simulink model "PV_MEV"  (R2025a)
settings: Solver=VariableStepAuto  StartTime=0.0  StopTime=10.0  RelTol=1e-3
InitFcn:
  | init_paras
values from neighbouring files (symbols this model uses):
  C_PFC = 2600e-6    (= 0.0026)    [init_paras.m]
  chg_ctrl_par = [Icc Vcv V_hys T_hys Kp_v_chg Ki_v_chg Kp_i_chg Ki_i_chg Ts_chg D_max_chg t_chg_on k_chg]    [init_paras.m]
  chg_ev = [0 Icc]    [init_paras.m]
  chg_par = [L_chg Voc Rint Ts_chg I_SIGN t_chg_on]    [init_paras.m]
  D = struct('X', {}, 'ti', {}, 'ia', {}, 'tc', {}, 'irms', {}, 'thd', {}, 'trip', {}, 'ttrip', {})    [make_waveform_figs.m]    (also in run_benchmark.m = get_sig('D'))
  det_ema_alpha = 0.1    [init_paras.m]
  det_force = 0    [init_paras.m]
  det_hyst = 0.6    [init_paras.m]
  det_persist = 2    [init_paras.m]
  det_src = 0    [init_paras.m]
  det_t_arm = 0.58    [init_paras.m]
  det_thr = [0.5 0.5 0.5 0.5 0.5]    [init_paras.m]
  det_variant_onehot = double(det_vlist == VARIANT_NAME)    [init_paras.m]
  ENABLE_HIL = 0    [init_paras.m]
  ENABLE_HIL_DET = 0    [init_paras.m]
  ENABLE_HIL_EST = 0    [init_paras.m]
  estimation_src = cfg_row.estimation_src    [init_paras.m]
  Fnom = 50    [init_paras.m]
  Fr_I = Fnom*2    (= 100)    [init_paras.m]
  grid_df = 0    [init_paras.m]
  grid_h5 = 0    [init_paras.m]
  grid_h7 = 0    [init_paras.m]
  grid_var_t0 = 0.7    [init_paras.m]
  hgq_fusion_alpha = [0.6704476522845647 0.7221651725151749 0.6446423751787858 0.41926421682656173]    [init_paras.m]
  hgq_min_ratio = single(0)    [init_paras.m]
  inj_channel = INJ.channel    [init_paras.m]
  inj_dwell = INJ.dwell    [init_paras.m]
  inj_shape = INJ.shape    [init_paras.m]
  inj_t_on = INJ.t_on    [init_paras.m]
  Ki_V = 80    [init_paras.m]
  Kp_I = 0.06    [init_paras.m]
  Kp_V = 0.25    [init_paras.m]
  Kr_I = 2.5    [init_paras.m]
  L_PFC = 600e-6    (= 0.0006)    [init_paras.m]
  Limit_V = 100    [init_paras.m]
  mit_t_ramp = 0.06    [init_paras.m]
  mitigation_mask = 0    [init_paras.m]
  mm_10cycle_points = mm_points_per_cycle * 10    (= 800)    [init_paras.m]
  mm_fund_freq = 50    [init_paras.m]
  mm_points_per_cycle = 80    [init_paras.m]
  R_bleed = 100e3    (= 100000)    [init_paras.m]
  R_pre = Ro*2    (= 44.44)    [init_paras.m]
  res_par = double(RES.par(:)'); end    [init_paras.m]
  RL_PFC = 20e-3    (= 0.02)    [init_paras.m]
  Ro = 22.22    [init_paras.m]
  t_pre_off = 0.30    (= 0.3)    [init_paras.m]
  Ts_chg = 10e-6    (= 1e-05)    [init_paras.m]
  Ts_Control = 1/Fc    [init_paras.m]
  Ts_Power = 50e-9    (= 5e-08)    [init_paras.m]    (also in run_benchmark.m = evalin('base','Ts_Power'))
  use_d_predict = cfg_row.use_d_predict    [init_paras.m]
  use_detector = 0    [init_paras.m]
  use_harmonic = cfg_row.use_harmonic    [init_paras.m]
  use_p_predict = cfg_row.use_p_predict    [init_paras.m]
  Vnom_ac = 240    [init_paras.m]
  vref_ev = [0 0]    [init_paras.m]
undefined symbols (not defined in the file or in its folder): D1, Delta, DiscIntNeverNeededParam
libraries: spsSeriesRLCBranchLib x17, spsMeanLib x16, MyLibrary x12, spsCurrentMeasurementLib x9, spsFourierLib x8, spsTHDLib x8, spsVoltageMeasurementLib x8, spsDiodeLib x7, simulink x7, pycoexlib x5, instrumentlib x4, spsPWMGeneratorDCDCLib x4
(part 3 of 7)

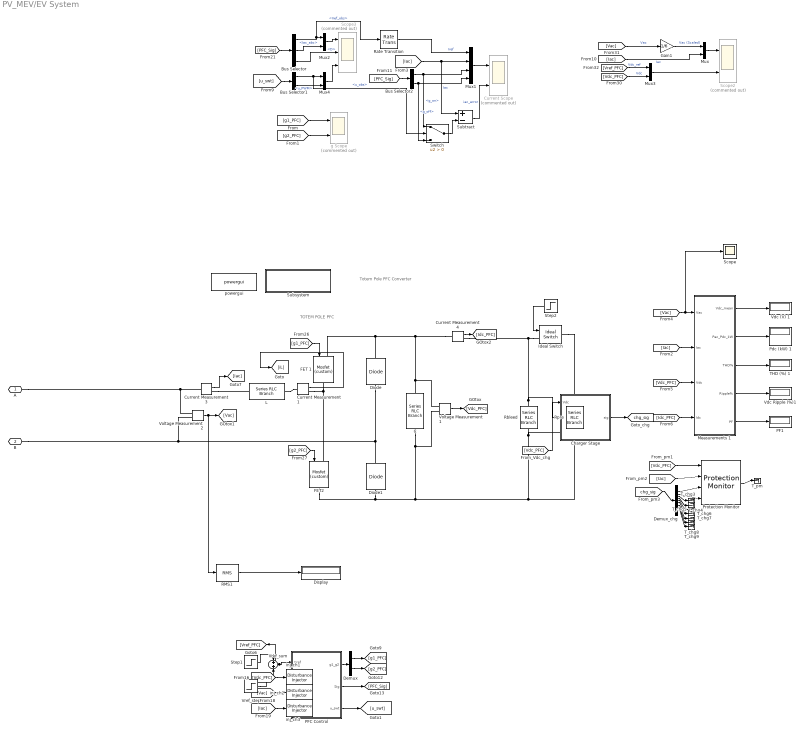
== system PV_MEV/EV System ==
  note: TOTEM POLE PFC
  note: Totem Pole PFC Converter
  Bus Selector : BusSelector  OutputSignals=Iref_obs,Iac_abc,D
  Bus Selector1 : BusSelector  OutputSignals=u_obs,u_PWM
  Bus Selector2 : BusSelector  OutputSignals=g_on,g_off
  C : spsSeriesRLCBranchLib/Series RLC Branch  LConnTagsString=__new0  RConnTagsString=__new0  BranchType=C  Resistance=1  Inductance=1e-3  SetiL0=off  InitialCurrent=0  Capacitance=C_PFC  Setx0=on  InitialVoltage=375  Measurements=None
  Charger Stage : Subsystem  mask(Charger Stage){}
      mask Display: disp('charger\\nbuck + battery\\nCC/CV')
  Current Measurement1 : spsCurrentMeasurementLib/Current Measurement  PhasorSimulation=off  OutputType=Complex  PSBequivalent=0
  Current Measurement3 : spsCurrentMeasurementLib/Current Measurement  PhasorSimulation=off  OutputType=Complex  PSBequivalent=0
  Current Measurement4 : spsCurrentMeasurementLib/Current Measurement  PhasorSimulation=off  OutputType=Complex  PSBequivalent=0
  Current Scope : Scope  Commented=on  NumInputPorts=2
      settings: ActiveDisplayYMinimum=-76.3871  ActiveDisplayYMaximum=79.5142  DataLoggingSaveFormat=Array
  Demux : Demux  Outputs=2
  Demux_chg : Demux  Outputs=9
  Diode : spsDiodeLib/Diode  Ron=Ron_Diode  Lon=0  Vf=Vf  IC=0  UseSnubber=0  Rs=1e6  Cs=inf  Measurements=off
  Diode1 : spsDiodeLib/Diode  Ron=Ron_Diode  Lon=0  Vf=Vf  IC=0  UseSnubber=0  Rs=1e6  Cs=inf  Measurements=off
  Display : Display
  FET 1 : MyLibrary/Mosfet (custom)  Ron=Ron_FET  Lon=0  Rd=Ron_Diode  Vfd=Vf  IC=0  Rs=1e6  Cs=inf  Measurements=off
  FET2 : MyLibrary/Mosfet (custom)  Ron=Ron_FET  Lon=0  Rd=Ron_Diode  Vfd=Vf  IC=0  Rs=1e6  Cs=inf  Measurements=off
  Gain1 : Gain  Gain=1/6
  Ideal Switch : spsIdealSwitchLib/Ideal Switch  Ron=0.001  Lon=0  IC=0  Rs=1e5  Cs=inf  Measurements=off
  L : spsSeriesRLCBranchLib/Series RLC Branch  LConnTagsString=__new0  RConnTagsString=__new0  BranchType=RL  Resistance=RL_PFC  Inductance=L_PFC  SetiL0=off  InitialCurrent=0  Capacitance=1e-6  Setx0=off  InitialVoltage=0  Measurements=None
  Measurements 1 : Subsystem
  Mux{,2..4} (4 alike) : Mux  Inputs=2
  Mux1 : Mux
  PF1 : Display
      settings: Format=bank  Decimation=100
  PFC Control : Subsystem
  Pdc (kW) 1 : Display
      settings: Format=bank  Decimation=100
  Protection Monitor : MyLibrary/Protection Monitor  SystemSampleTime=-1  VariantActivationTime=update diagram  EmptyChoice=off  PassThrough=off  PassThroughVariantControl=(default)  EmptyChoiceVariantControl=(default)  AllowFlexibleInterface=on  Latency=0  AutoFrameSizeCalculation=off
  RMS1 : spsRMSLib/RMS  TrueRMS=on  Freq=60  RMSInit=0  Ts=5E-08
  Rate Transition : RateTransition
  Rbleed : spsSeriesRLCBranchLib/Series RLC Branch  LConnTagsString=__new0  RConnTagsString=__new0  BranchType=R  Resistance=R_bleed  Inductance=200e-6  SetiL0=off  InitialCurrent=0  Capacitance=400e-6  Setx0=off  InitialVoltage=0  Measurements=None
  Rpre : spsSeriesRLCBranchLib/Series RLC Branch  LConnTagsString=__new0  RConnTagsString=__new0  BranchType=R  Resistance=R_pre  Inductance=200e-6  SetiL0=off  InitialCurrent=0  Capacitance=400e-6  Setx0=off  InitialVoltage=0  Measurements=None
  Scope : Scope
      settings: ActiveDisplayYMaximum=209.9376  DataLoggingVariableName=ScopeData2  DataLoggingSaveFormat=Array
  Scope2 : Scope  Commented=on  NumInputPorts=2
      settings: ActiveDisplayYMinimum=-127.2219  ActiveDisplayYMaximum=127.2109  DataLoggingVariableName=ScopeData3  DataLoggingSaveFormat=Array
  Scope3 : Scope  Commented=on  NumInputPorts=3
      settings: ActiveDisplayYMinimum=-13.4274  ActiveDisplayYMaximum=110.8467  DataLoggingVariableName=ScopeData4  DataLoggingSaveFormat=Array
  Step1 : Step  Time=0.2  Before=350  After=400  SampleTime=Ts_Power
  Step2 : Step  Time=t_pre_off  Before=1  After=0  SampleTime=Ts_Power
  Subsystem : Subsystem
      settings: OpenFcn=edit('Totem_Pole_PFC_v1_data');
      mask Display: disp('Double-click to open\n parameters file');
  Subtract : Sum  Inputs=+-
  Switch : Switch  Criteria=u2 > Threshold  SaturateOnIntegerOverflow=off  InputSameDT=off
  THD (%) 1 : Display
      settings: Format=bank  Decimation=100
  T_chg{3..9} (7 alike) : Terminator
  T_pm : Terminator
  Vdc (V) 1 : Display
      settings: Format=bank  Decimation=100
  Vdc Ripple (%)1 : Display
      settings: Format=bank  Decimation=100
  Voltage Measurement1 : spsVoltageMeasurementLib/Voltage Measurement  PhasorSimulation=off  OutputType=Complex  PSBequivalent=0
  Voltage Measurement2 : spsVoltageMeasurementLib/Voltage Measurement  PhasorSimulation=off  OutputType=Complex  PSBequivalent=0
  Vref_step : Step  Time=vref_ev(1)  After=vref_ev(2)  SampleTime=0
  Vref_sum : Sum
  g Scope : Scope  Commented=on  NumInputPorts=2
      settings: ActiveDisplayYMinimum=-0.125  ActiveDisplayYMaximum=1.125  DataLoggingVariableName=ScopeData5  DataLoggingSaveFormat=Array
  inj_ch1 : MyLibrary/Disturbance Injector  ch_id=1  Ts_inj=Ts_Control  Ts_out=Ts_Power
  inj_ch2 : MyLibrary/Disturbance Injector  ch_id=2  Ts_inj=Ts_Control  Ts_out=Ts_Power
  inj_ch3 : MyLibrary/Disturbance Injector  ch_id=3  Ts_inj=Ts_Control  Ts_out=Ts_Power
  powergui : spspowerguiLib/powergui  Priority=1  SimulationMode=Discrete  SampleTime=Ts_Power  frequency=60  Iterations=50  frequencyindice=0  Pbase=100e6  ErrMax=1e-4  UnitsV=kV  UnitsW=MW  buscounter=0  FunctionMessages=off  echomessages=off  EnableUseOfTLC=off  CurrentSourceSwitches=off  DisableSnubberDevices=off  DisableRonSwitches=off  DisableVfSwitches=off  DisplayEquations=off  AutomaticDiscreteSolvers=off  SolverType=Tustin/Backward Euler (TBE)  Interpol=off  ExternalGateDelay=off  methode=off  Ts=100  x0status=blocks  SPID=on  SwTol=0  HookPort=off  NonlinearTolerance=1e-4  nMaxIteration=100  ContinueOnMaxIteration=off  RestoreLinks=warning  ResistiveCurrentMeasurement=off  Frange=[0:2:500]  Ylog=off  Xlog=on  ShowGrid=off  save=off  variable=ZData  structure=0  ZoomFFT=off  StartTime=0.0  cycles=1  DisplayStyle=1  fundamental=60  FreqAxis=off  MaxFrequency=1000  frequencyindicesteady=1  RmsSteady=1  display=off
  A : PMIOPort  Side=Left
  B : PMIOPort  Port=2  Side=Left
  tag scope: chg_sig=global
  wires:
  Bus Selector1/1 -> Mux4/1, Switch/2  "<u_obs>"
  Bus Selector/2 -> Mux2/2  "<Iac_abc>"
  [g2_PFC] -> FET2/1
  [Iac] -> Measurements 1/2(Iac)
  Bus Selector/3 -> Scope3/2  "<D>"
  [g1_PFC] -> g Scope/1
  Measurements 1/3(THD%) -> THD (%) 1/1
  Voltage Measurement2/1 -> RMS1/1, [Vac]
  Mux3/1 -> Scope2/2
  Measurements 1/4(Ripple%) -> Vdc Ripple (%)1/1
  PFC Control/1(g1_g2) -> Demux/1
  PFC Control/3(u_swt) -> [u_swt]
  Bus Selector2/2 -> Mux1/4, Switch/3  "<g_off>"
  Mux2/1 -> Scope3/1
  Measurements 1/2(Pac_Pdc_kW) -> Pdc (kW) 1/1
  Step2/1 -> Ideal Switch/1
  [Idc_PFC] -> Measurements 1/4(Idc)
  [Iac] -> Subtract/1, Mux1/2  "Iac"
  Gain1/1 -> Mux/1  "Vac (Scaled)"
  [u_swt] -> Bus Selector1/1
  Bus Selector/1 -> Rate Transition/1, Mux2/1  "<Iref_obs>"
  Measurements 1/1(Vdc_mean) -> Vdc (V) 1/1
  [g2_PFC] -> g Scope/2
  [PFC_Sig] -> Bus Selector2/1
  [Vac] -> Scope/1, Measurements 1/1(Vac)
  [Vac] -> Gain1/1  "Vac"
  PFC Control/2(Sig) -> [PFC_Sig]
  [PFC_Sig] -> Bus Selector/1
  Voltage Measurement1/1 -> [Vdc_PFC]
  [g1_PFC] -> FET 1/1
  [Vdc_PFC] -> Measurements 1/3(Vdc)
  Mux/1 -> Scope2/1
  Bus Selector1/2 -> Mux4/2  "<u_PWM>"
  RMS1/1 -> Display/1
  Current Measurement3/1 -> [Iac]
  [Iac] -> Mux/2  "Iac"
  Bus Selector2/1 -> Switch/1, Mux1/3  "<g_on>"
  Switch/1 -> Subtract/2
  Current Measurement1/1 -> [iL]
  Mux4/1 -> Scope3/3
  [Vdc_PFC] -> Mux3/2  "Vdc"
  Demux/1 -> [g1_PFC]
  Demux/2 -> [g2_PFC]
  Rate Transition/1 -> Mux1/1  "Iref"
  Measurements 1/5(PF) -> PF1/1
  Mux1/1 -> Current Scope/1
  [Vref_PFC] -> Mux3/1  "Vdc_ref"
  Subtract/1 -> Current Scope/2  "iac_error"
  Current Measurement4/1 -> [Idc_PFC]
  [Vdc_PFC] -> Charger Stage/1(Vdc)
  Charger Stage/1(sig) -> [chg_sig]
  [Vdc_PFC] -> inj_ch1/1
  inj_ch1/1 -> PFC Control/2(Vdc)
  [Vac] -> inj_ch2/1
  inj_ch2/1 -> PFC Control/3(Vac)
  [Iac] -> inj_ch3/1
  inj_ch3/1 -> PFC Control/4(Iac)
  [Vdc_PFC] -> Protection Monitor/1
  [Iac] -> Protection Monitor/2
  [chg_sig] -> Demux_chg/1
  Demux_chg/1 -> Protection Monitor/3
  Demux_chg/2 -> Protection Monitor/4
  Demux_chg/3 -> T_chg3/1
  Demux_chg/4 -> T_chg4/1
  Demux_chg/5 -> T_chg5/1
  Demux_chg/6 -> T_chg6/1
  Demux_chg/7 -> T_chg7/1
  Demux_chg/8 -> T_chg8/1
  Demux_chg/9 -> T_chg9/1
  Protection Monitor/1 -> T_pm/1
  Step1/1 -> Vref_sum/1
  Vref_step/1 -> Vref_sum/2
  Vref_sum/1 -> PFC Control/1(Vref), [Vref_PFC]
  connections:
  Ideal Switch/LConn1 -- Current Measurement4/RConn1 -- Rbleed/LConn1 -- Charger Stage/LConn1
  Current Measurement1/RConn1 -- FET2/LConn1 -- FET 1/RConn1
  Rpre/RConn1 -- Rbleed/RConn1 -- Charger Stage/LConn2 -- C/RConn1 -- Voltage Measurement1/LConn2 -- FET2/RConn1 -- Diode1/LConn1
  Voltage Measurement2/LConn2 -- B/RConn1 -- Diode/LConn1 -- Diode1/RConn1
  Current Measurement4/LConn1 -- Voltage Measurement1/LConn1 -- C/LConn1 -- Diode/RConn1 -- FET 1/LConn1
  Voltage Measurement2/LConn1 -- A/RConn1 -- Current Measurement3/LConn1
  Current Measurement3/RConn1 -- L/LConn1
  L/RConn1 -- Current Measurement1/LConn1
  Ideal Switch/RConn1 -- Rpre/LConn1

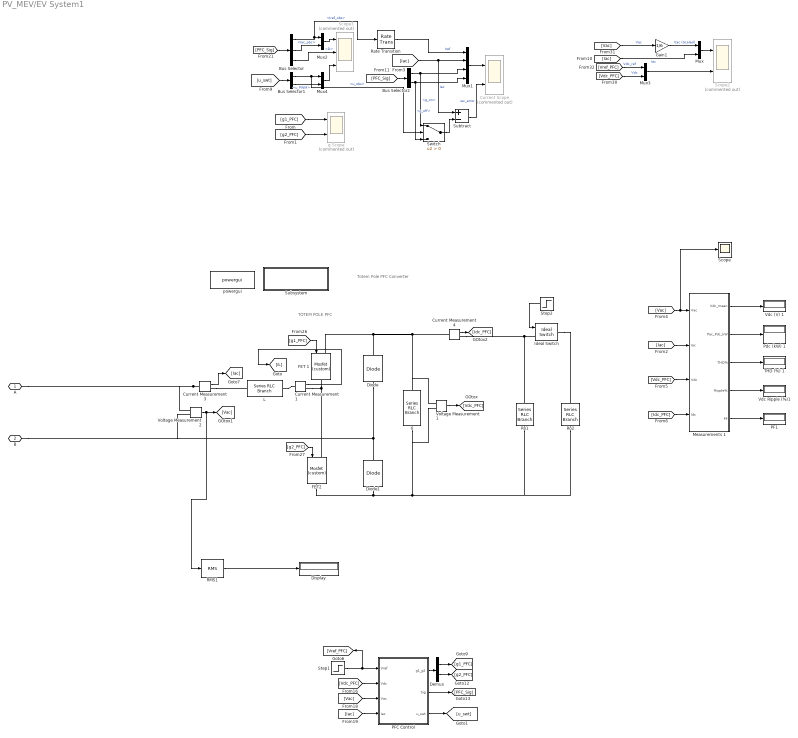
== system PV_MEV/EV System1 ==
  note: Totem Pole PFC Converter
  note: TOTEM POLE PFC
  Bus Selector : BusSelector  OutputSignals=Iref_obs,Iac_abc,D
  Bus Selector1 : BusSelector  OutputSignals=u_obs,u_PWM
  Bus Selector2 : BusSelector  OutputSignals=g_on,g_off
  C : spsSeriesRLCBranchLib/Series RLC Branch  LConnTagsString=__new0  RConnTagsString=__new0  BranchType=C  Resistance=1  Inductance=1e-3  SetiL0=off  InitialCurrent=0  Capacitance=C_PFC  Setx0=on  InitialVoltage=375  Measurements=None
  Current Measurement1 : spsCurrentMeasurementLib/Current Measurement  PhasorSimulation=off  OutputType=Complex  PSBequivalent=0
  Current Measurement3 : spsCurrentMeasurementLib/Current Measurement  PhasorSimulation=off  OutputType=Complex  PSBequivalent=0
  Current Measurement4 : spsCurrentMeasurementLib/Current Measurement  PhasorSimulation=off  OutputType=Complex  PSBequivalent=0
  Current Scope : Scope  Commented=on  NumInputPorts=2
      settings: ActiveDisplayYMinimum=-76.3871  ActiveDisplayYMaximum=79.5142  DataLoggingSaveFormat=Array
  Demux : Demux  Outputs=2
  Diode : spsDiodeLib/Diode  Ron=Ron_Diode  Lon=0  Vf=Vf  IC=0  UseSnubber=0  Rs=1e6  Cs=inf  Measurements=off
  Diode1 : spsDiodeLib/Diode  Ron=Ron_Diode  Lon=0  Vf=Vf  IC=0  UseSnubber=0  Rs=1e6  Cs=inf  Measurements=off
  Display : Display
  FET 1 : MyLibrary/Mosfet (custom)  Ron=Ron_FET  Lon=0  Rd=Ron_Diode  Vfd=Vf  IC=0  Rs=1e6  Cs=inf  Measurements=off
  FET2 : MyLibrary/Mosfet (custom)  Ron=Ron_FET  Lon=0  Rd=Ron_Diode  Vfd=Vf  IC=0  Rs=1e6  Cs=inf  Measurements=off
  Gain1 : Gain  Gain=1/6
  Ideal Switch : spsIdealSwitchLib/Ideal Switch  Ron=0.001  Lon=0  IC=0  Rs=1e5  Cs=inf  Measurements=off
  L : spsSeriesRLCBranchLib/Series RLC Branch  LConnTagsString=__new0  RConnTagsString=__new0  BranchType=RL  Resistance=RL_PFC  Inductance=L_PFC  SetiL0=off  InitialCurrent=0  Capacitance=1e-6  Setx0=off  InitialVoltage=0  Measurements=None
  Measurements 1 : Subsystem
  Mux{,2..4} (4 alike) : Mux  Inputs=2
  Mux1 : Mux
  PF1 : Display
      settings: Format=bank  Decimation=100
  PFC Control : Subsystem
  Pdc (kW) 1 : Display
      settings: Format=bank  Decimation=100
  RMS1 : spsRMSLib/RMS  TrueRMS=on  Freq=60  RMSInit=0  Ts=5E-08
  Rate Transition : RateTransition
  Ro1 : spsSeriesRLCBranchLib/Series RLC Branch  LConnTagsString=__new0  RConnTagsString=__new0  BranchType=R  Resistance=Ro*2  Inductance=200e-6  SetiL0=off  InitialCurrent=0  Capacitance=400e-6  Setx0=off  InitialVoltage=0  Measurements=None
  Ro2 : spsSeriesRLCBranchLib/Series RLC Branch  LConnTagsString=__new0  RConnTagsString=__new0  BranchType=R  Resistance=Ro*2  Inductance=200e-6  SetiL0=off  InitialCurrent=0  Capacitance=400e-6  Setx0=off  InitialVoltage=0  Measurements=None
  Scope : Scope
      settings: DataLoggingVariableName=ScopeData2  DataLoggingSaveFormat=Array
  Scope2 : Scope  Commented=on  NumInputPorts=2
      settings: ActiveDisplayYMinimum=-127.2219  ActiveDisplayYMaximum=127.2109  DataLoggingVariableName=ScopeData3  DataLoggingSaveFormat=Array
  Scope3 : Scope  Commented=on  NumInputPorts=3
      settings: ActiveDisplayYMinimum=-13.4274  ActiveDisplayYMaximum=110.8467  DataLoggingVariableName=ScopeData4  DataLoggingSaveFormat=Array
  Step1 : Step  Time=0.2  Before=350  After=400  SampleTime=Ts_Power
  Step2 : Step  Time=0.4  SampleTime=Ts_Power
  Subsystem : Subsystem
      settings: OpenFcn=edit('Totem_Pole_PFC_v1_data');
      mask Display: disp('Double-click to open\n parameters file');
  Subtract : Sum  Inputs=+-
  Switch : Switch  Criteria=u2 > Threshold  SaturateOnIntegerOverflow=off  InputSameDT=off
  THD (%) 1 : Display
      settings: Format=bank  Decimation=100
  Vdc (V) 1 : Display
      settings: Format=bank  Decimation=100
  Vdc Ripple (%)1 : Display
      settings: Format=bank  Decimation=100
  Voltage Measurement1 : spsVoltageMeasurementLib/Voltage Measurement  PhasorSimulation=off  OutputType=Complex  PSBequivalent=0
  Voltage Measurement2 : spsVoltageMeasurementLib/Voltage Measurement  PhasorSimulation=off  OutputType=Complex  PSBequivalent=0
  g Scope : Scope  Commented=on  NumInputPorts=2
      settings: ActiveDisplayYMinimum=-0.125  ActiveDisplayYMaximum=1.125  DataLoggingVariableName=ScopeData5  DataLoggingSaveFormat=Array
  powergui : spspowerguiLib/powergui  Priority=1  SimulationMode=Discrete  SampleTime=Ts_Power  frequency=60  Iterations=50  frequencyindice=0  Pbase=100e6  ErrMax=1e-4  UnitsV=kV  UnitsW=MW  buscounter=0  FunctionMessages=off  echomessages=off  EnableUseOfTLC=off  CurrentSourceSwitches=off  DisableSnubberDevices=off  DisableRonSwitches=off  DisableVfSwitches=off  DisplayEquations=off  AutomaticDiscreteSolvers=off  SolverType=Tustin/Backward Euler (TBE)  Interpol=off  ExternalGateDelay=off  methode=off  Ts=100  x0status=blocks  SPID=on  SwTol=0  HookPort=off  NonlinearTolerance=1e-4  nMaxIteration=100  ContinueOnMaxIteration=off  RestoreLinks=warning  ResistiveCurrentMeasurement=off  Frange=[0:2:500]  Ylog=off  Xlog=on  ShowGrid=off  save=off  variable=ZData  structure=0  ZoomFFT=off  StartTime=0.0  cycles=1  DisplayStyle=1  fundamental=60  FreqAxis=off  MaxFrequency=1000  frequencyindicesteady=1  RmsSteady=1  display=off
  A : PMIOPort  Side=Left
  B : PMIOPort  Port=2  Side=Left
  wires:
  Current Measurement4/1 -> [Idc_PFC]
  Subtract/1 -> Current Scope/2  "iac_error"
  [Vref_PFC] -> Mux3/1  "Vdc_ref"
  Mux1/1 -> Current Scope/1
  Measurements 1/5(PF) -> PF1/1
  Rate Transition/1 -> Mux1/1  "Iref"
  Demux/2 -> [g2_PFC]
  Demux/1 -> [g1_PFC]
  [Vdc_PFC] -> Mux3/2  "Vdc"
  Mux4/1 -> Scope3/3
  [Iac] -> PFC Control/4(Iac)
  Current Measurement1/1 -> [iL]
  Switch/1 -> Subtract/2
  Bus Selector2/1 -> Mux1/3, Switch/1  "<g_on>"
  [Iac] -> Mux/2  "Iac"
  Current Measurement3/1 -> [Iac]
  RMS1/1 -> Display/1
  Bus Selector1/2 -> Mux4/2  "<u_PWM>"
  Mux/1 -> Scope2/1
  [Vdc_PFC] -> Measurements 1/3(Vdc)
  [Vac] -> PFC Control/3(Vac)
  [g1_PFC] -> FET 1/1
  Voltage Measurement1/1 -> [Vdc_PFC]
  [Vdc_PFC] -> PFC Control/2(Vdc)
  [PFC_Sig] -> Bus Selector/1
  PFC Control/2(Sig) -> [PFC_Sig]
  [Vac] -> Gain1/1  "Vac"
  [Vac] -> Measurements 1/1(Vac), Scope/1
  [PFC_Sig] -> Bus Selector2/1
  [g2_PFC] -> g Scope/2
  Measurements 1/1(Vdc_mean) -> Vdc (V) 1/1
  Bus Selector/1 -> Mux2/1, Rate Transition/1  "<Iref_obs>"
  [u_swt] -> Bus Selector1/1
  Gain1/1 -> Mux/1  "Vac (Scaled)"
  [Iac] -> Mux1/2, Subtract/1  "Iac"
  [Idc_PFC] -> Measurements 1/4(Idc)
  Step2/1 -> Ideal Switch/1
  Measurements 1/2(Pac_Pdc_kW) -> Pdc (kW) 1/1
  Mux2/1 -> Scope3/1
  Bus Selector2/2 -> Switch/3, Mux1/4  "<g_off>"
  PFC Control/3(u_swt) -> [u_swt]
  PFC Control/1(g1_g2) -> Demux/1
  Measurements 1/4(Ripple%) -> Vdc Ripple (%)1/1
  Mux3/1 -> Scope2/2
  Voltage Measurement2/1 -> [Vac], RMS1/1
  Measurements 1/3(THD%) -> THD (%) 1/1
  [g1_PFC] -> g Scope/1
  Bus Selector/3 -> Scope3/2  "<D>"
  [Iac] -> Measurements 1/2(Iac)
  [g2_PFC] -> FET2/1
  Step1/1 -> [Vref_PFC], PFC Control/1(Vref)
  Bus Selector/2 -> Mux2/2  "<Iac_abc>"
  Bus Selector1/1 -> Switch/2, Mux4/1  "<u_obs>"
  connections:
  Ideal Switch/RConn1 -- Ro2/LConn1
  L/RConn1 -- Current Measurement1/LConn1
  Current Measurement3/RConn1 -- L/LConn1
  Current Measurement3/LConn1 -- A/RConn1 -- Voltage Measurement2/LConn1
  FET 1/LConn1 -- Diode/RConn1 -- C/LConn1 -- Voltage Measurement1/LConn1 -- Current Measurement4/LConn1
  Diode1/RConn1 -- Diode/LConn1 -- B/RConn1 -- Voltage Measurement2/LConn2
  Diode1/LConn1 -- FET2/RConn1 -- Voltage Measurement1/LConn2 -- C/RConn1 -- Ro1/RConn1 -- Ro2/RConn1
  FET 1/RConn1 -- FET2/LConn1 -- Current Measurement1/RConn1
  Current Measurement4/RConn1 -- Ro1/LConn1 -- Ideal Switch/LConn1

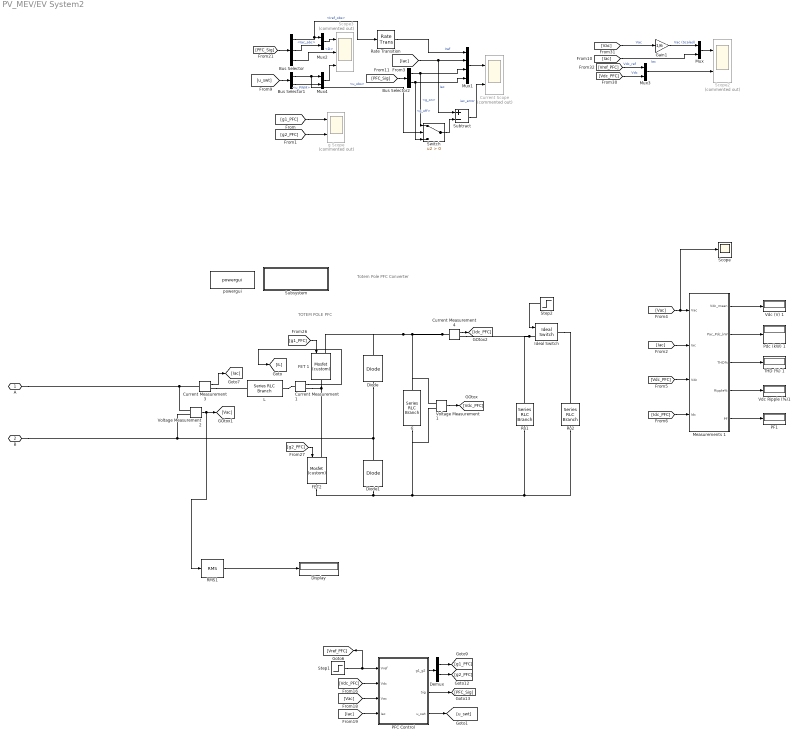
== system PV_MEV/EV System2 ==
  note: TOTEM POLE PFC
  note: Totem Pole PFC Converter
  Bus Selector : BusSelector  OutputSignals=Iref_obs,Iac_abc,D
  Bus Selector1 : BusSelector  OutputSignals=u_obs,u_PWM
  Bus Selector2 : BusSelector  OutputSignals=g_on,g_off
  C : spsSeriesRLCBranchLib/Series RLC Branch  LConnTagsString=__new0  RConnTagsString=__new0  BranchType=C  Resistance=1  Inductance=1e-3  SetiL0=off  InitialCurrent=0  Capacitance=C_PFC  Setx0=on  InitialVoltage=375  Measurements=None
  Current Measurement1 : spsCurrentMeasurementLib/Current Measurement  PhasorSimulation=off  OutputType=Complex  PSBequivalent=0
  Current Measurement3 : spsCurrentMeasurementLib/Current Measurement  PhasorSimulation=off  OutputType=Complex  PSBequivalent=0
  Current Measurement4 : spsCurrentMeasurementLib/Current Measurement  PhasorSimulation=off  OutputType=Complex  PSBequivalent=0
  Current Scope : Scope  Commented=on  NumInputPorts=2
      settings: ActiveDisplayYMinimum=-76.3871  ActiveDisplayYMaximum=79.5142  DataLoggingSaveFormat=Array
  Demux : Demux  Outputs=2
  Diode : spsDiodeLib/Diode  Ron=Ron_Diode  Lon=0  Vf=Vf  IC=0  UseSnubber=0  Rs=1e6  Cs=inf  Measurements=off
  Diode1 : spsDiodeLib/Diode  Ron=Ron_Diode  Lon=0  Vf=Vf  IC=0  UseSnubber=0  Rs=1e6  Cs=inf  Measurements=off
  Display : Display
  FET 1 : MyLibrary/Mosfet (custom)  Ron=Ron_FET  Lon=0  Rd=Ron_Diode  Vfd=Vf  IC=0  Rs=1e6  Cs=inf  Measurements=off
  FET2 : MyLibrary/Mosfet (custom)  Ron=Ron_FET  Lon=0  Rd=Ron_Diode  Vfd=Vf  IC=0  Rs=1e6  Cs=inf  Measurements=off
  Gain1 : Gain  Gain=1/6
  Ideal Switch : spsIdealSwitchLib/Ideal Switch  Ron=0.001  Lon=0  IC=0  Rs=1e5  Cs=inf  Measurements=off
  L : spsSeriesRLCBranchLib/Series RLC Branch  LConnTagsString=__new0  RConnTagsString=__new0  BranchType=RL  Resistance=RL_PFC  Inductance=L_PFC  SetiL0=off  InitialCurrent=0  Capacitance=1e-6  Setx0=off  InitialVoltage=0  Measurements=None
  Measurements 1 : Subsystem
  Mux{,2..4} (4 alike) : Mux  Inputs=2
  Mux1 : Mux
  PF1 : Display
      settings: Format=bank  Decimation=100
  PFC Control : Subsystem
  Pdc (kW) 1 : Display
      settings: Format=bank  Decimation=100
  RMS1 : spsRMSLib/RMS  TrueRMS=on  Freq=60  RMSInit=0  Ts=5E-08
  Rate Transition : RateTransition
  Ro1 : spsSeriesRLCBranchLib/Series RLC Branch  LConnTagsString=__new0  RConnTagsString=__new0  BranchType=R  Resistance=Ro*2  Inductance=200e-6  SetiL0=off  InitialCurrent=0  Capacitance=400e-6  Setx0=off  InitialVoltage=0  Measurements=None
  Ro2 : spsSeriesRLCBranchLib/Series RLC Branch  LConnTagsString=__new0  RConnTagsString=__new0  BranchType=R  Resistance=Ro*2  Inductance=200e-6  SetiL0=off  InitialCurrent=0  Capacitance=400e-6  Setx0=off  InitialVoltage=0  Measurements=None
  Scope : Scope
      settings: DataLoggingVariableName=ScopeData2  DataLoggingSaveFormat=Array
  Scope2 : Scope  Commented=on  NumInputPorts=2
      settings: ActiveDisplayYMinimum=-127.2219  ActiveDisplayYMaximum=127.2109  DataLoggingVariableName=ScopeData3  DataLoggingSaveFormat=Array
  Scope3 : Scope  Commented=on  NumInputPorts=3
      settings: ActiveDisplayYMinimum=-13.4274  ActiveDisplayYMaximum=110.8467  DataLoggingVariableName=ScopeData4  DataLoggingSaveFormat=Array
  Step1 : Step  Time=0.2  Before=350  After=400  SampleTime=Ts_Power
  Step2 : Step  Time=0.4  SampleTime=Ts_Power
  Subsystem : Subsystem
      settings: OpenFcn=edit('Totem_Pole_PFC_v1_data');
      mask Display: disp('Double-click to open\n parameters file');
  Subtract : Sum  Inputs=+-
  Switch : Switch  Criteria=u2 > Threshold  SaturateOnIntegerOverflow=off  InputSameDT=off
  THD (%) 1 : Display
      settings: Format=bank  Decimation=100
  Vdc (V) 1 : Display
      settings: Format=bank  Decimation=100
  Vdc Ripple (%)1 : Display
      settings: Format=bank  Decimation=100
  Voltage Measurement1 : spsVoltageMeasurementLib/Voltage Measurement  PhasorSimulation=off  OutputType=Complex  PSBequivalent=0
  Voltage Measurement2 : spsVoltageMeasurementLib/Voltage Measurement  PhasorSimulation=off  OutputType=Complex  PSBequivalent=0
  g Scope : Scope  Commented=on  NumInputPorts=2
      settings: ActiveDisplayYMinimum=-0.125  ActiveDisplayYMaximum=1.125  DataLoggingVariableName=ScopeData5  DataLoggingSaveFormat=Array
  powergui : spspowerguiLib/powergui  Priority=1  SimulationMode=Discrete  SampleTime=Ts_Power  frequency=60  Iterations=50  frequencyindice=0  Pbase=100e6  ErrMax=1e-4  UnitsV=kV  UnitsW=MW  buscounter=0  FunctionMessages=off  echomessages=off  EnableUseOfTLC=off  CurrentSourceSwitches=off  DisableSnubberDevices=off  DisableRonSwitches=off  DisableVfSwitches=off  DisplayEquations=off  AutomaticDiscreteSolvers=off  SolverType=Tustin/Backward Euler (TBE)  Interpol=off  ExternalGateDelay=off  methode=off  Ts=100  x0status=blocks  SPID=on  SwTol=0  HookPort=off  NonlinearTolerance=1e-4  nMaxIteration=100  ContinueOnMaxIteration=off  RestoreLinks=warning  ResistiveCurrentMeasurement=off  Frange=[0:2:500]  Ylog=off  Xlog=on  ShowGrid=off  save=off  variable=ZData  structure=0  ZoomFFT=off  StartTime=0.0  cycles=1  DisplayStyle=1  fundamental=60  FreqAxis=off  MaxFrequency=1000  frequencyindicesteady=1  RmsSteady=1  display=off
  A : PMIOPort  Side=Left
  B : PMIOPort  Port=2  Side=Left
  wires:
  Bus Selector1/1 -> Mux4/1, Switch/2  "<u_obs>"
  Bus Selector/2 -> Mux2/2  "<Iac_abc>"
  Step1/1 -> PFC Control/1(Vref), [Vref_PFC]
  [g2_PFC] -> FET2/1
  [Iac] -> Measurements 1/2(Iac)
  Bus Selector/3 -> Scope3/2  "<D>"
  [g1_PFC] -> g Scope/1
  Measurements 1/3(THD%) -> THD (%) 1/1
  Voltage Measurement2/1 -> RMS1/1, [Vac]
  Mux3/1 -> Scope2/2
  Measurements 1/4(Ripple%) -> Vdc Ripple (%)1/1
  PFC Control/1(g1_g2) -> Demux/1
  PFC Control/3(u_swt) -> [u_swt]
  Bus Selector2/2 -> Mux1/4, Switch/3  "<g_off>"
  Mux2/1 -> Scope3/1
  Measurements 1/2(Pac_Pdc_kW) -> Pdc (kW) 1/1
  Step2/1 -> Ideal Switch/1
  [Idc_PFC] -> Measurements 1/4(Idc)
  [Iac] -> Subtract/1, Mux1/2  "Iac"
  Gain1/1 -> Mux/1  "Vac (Scaled)"
  [u_swt] -> Bus Selector1/1
  Bus Selector/1 -> Rate Transition/1, Mux2/1  "<Iref_obs>"
  Measurements 1/1(Vdc_mean) -> Vdc (V) 1/1
  [g2_PFC] -> g Scope/2
  [PFC_Sig] -> Bus Selector2/1
  [Vac] -> Scope/1, Measurements 1/1(Vac)
  [Vac] -> Gain1/1  "Vac"
  PFC Control/2(Sig) -> [PFC_Sig]
  [PFC_Sig] -> Bus Selector/1
  [Vdc_PFC] -> PFC Control/2(Vdc)
  Voltage Measurement1/1 -> [Vdc_PFC]
  [g1_PFC] -> FET 1/1
  [Vac] -> PFC Control/3(Vac)
  [Vdc_PFC] -> Measurements 1/3(Vdc)
  Mux/1 -> Scope2/1
  Bus Selector1/2 -> Mux4/2  "<u_PWM>"
  RMS1/1 -> Display/1
  Current Measurement3/1 -> [Iac]
  [Iac] -> Mux/2  "Iac"
  Bus Selector2/1 -> Switch/1, Mux1/3  "<g_on>"
  Switch/1 -> Subtract/2
  Current Measurement1/1 -> [iL]
  [Iac] -> PFC Control/4(Iac)
  Mux4/1 -> Scope3/3
  [Vdc_PFC] -> Mux3/2  "Vdc"
  Demux/1 -> [g1_PFC]
  Demux/2 -> [g2_PFC]
  Rate Transition/1 -> Mux1/1  "Iref"
  Measurements 1/5(PF) -> PF1/1
  Mux1/1 -> Current Scope/1
  [Vref_PFC] -> Mux3/1  "Vdc_ref"
  Subtract/1 -> Current Scope/2  "iac_error"
  Current Measurement4/1 -> [Idc_PFC]
  connections:
  Ideal Switch/LConn1 -- Ro1/LConn1 -- Current Measurement4/RConn1
  Current Measurement1/RConn1 -- FET2/LConn1 -- FET 1/RConn1
  Ro2/RConn1 -- Ro1/RConn1 -- C/RConn1 -- Voltage Measurement1/LConn2 -- FET2/RConn1 -- Diode1/LConn1
  Voltage Measurement2/LConn2 -- B/RConn1 -- Diode/LConn1 -- Diode1/RConn1
  Current Measurement4/LConn1 -- Voltage Measurement1/LConn1 -- C/LConn1 -- Diode/RConn1 -- FET 1/LConn1
  Voltage Measurement2/LConn1 -- A/RConn1 -- Current Measurement3/LConn1
  Current Measurement3/RConn1 -- L/LConn1
  L/RConn1 -- Current Measurement1/LConn1
  Ideal Switch/RConn1 -- Ro2/LConn1

== system PV_MEV/PV System ==
  note: 100-kW  PV Array
      | 330 * SunPower SPR-305E-WHT-D  (Nser=5 Npar=66)
  10 kvar : spsThreePhaseSeriesRLCLoadLib/Three-Phase Series RLC Load  LConnTagsString=A|B|C  Configuration=Y (grounded)  NominalVoltage=Vnom_ac  Vabc=[1e3 1e3 1e3]  Vabcp=[1e3 1e3 1e3]  NominalFrequency=Fnom  UnbalancedPower=off  ActivePower=10e3/100  InductivePower=0  CapacitivePower=10e3  Pabc=[10e3 9e3 11e3]  QLabc=[100 90 110]  QCabc=[100 90 110]  Pabcp=[10e3 9e3 11e3]  QLabcp=[100 90 110]  QCabcp=[100 90 110]  Measurements=None  LoadType=constant Z
  DC AC Inverter : Subsystem
  DC DC Boost Converter : Subsystem
  L : spsThreePhaseSeriesRLCBranchLib/Three-Phase Series RLC Branch  LConnTagsString=A|B|C  RConnTagsString=A|B|C  BranchType=RL  Resistance=500e-6*377/50/2  Inductance=500e-6/2  Capacitance=inf  Measurements=None
  PV Array : spsPVArrayLib/PV Array  Npar=66  Nser=5  PlotType=array @ 1000 W/m2 & specified temperatures  S_vec="[ 1000  250 ]"  Temp_C_vec="[0 25 50  ]"  ModuleName=SunPower SPR-305E-WHT-D  PlotWhenSelected=off  Pm=305.226  Ncell=96  Voc=64.2  Isc=5.96  Vm=54.7  Im=5.58  beta_Voc_pc=-0.2727  alpha_Isc_pc=0.061745  beta_Voc=-0.17507  alpha_Isc=0.00368  IL=5.9657  I0=6.3076e-12  nI=0.94489  Rsh=393.2054  Rs=0.37428  RobustModel=off  RobustCellTemperature=25  BAL=on  Tc=1e-6  Tfilter=5e-5
  PV Enviroment : Subsystem
  PV Status : Subsystem
  A : PMIOPort  Side=Right
  B : PMIOPort  Port=2  Side=Right
  C : PMIOPort  Port=3  Side=Right
  wires:
  PV Array/1 -> PV Status/1(m_PV)
  PV Enviroment/2(Temp) -> PV Array/2
  PV Enviroment/1(Ir) -> PV Array/1
  connections:
  10 kvar/LConn1 -- A/RConn1 -- L/RConn1
  10 kvar/LConn2 -- B/RConn1 -- L/RConn2
  10 kvar/LConn3 -- C/RConn1 -- L/RConn3
  DC AC Inverter/LConn1 -- DC DC Boost Converter/RConn1
  DC AC Inverter/LConn3 -- DC DC Boost Converter/RConn3
  DC AC Inverter/RConn3 -- L/LConn3
  DC AC Inverter/RConn2 -- L/LConn2
  PV Array/RConn1 -- DC DC Boost Converter/LConn1
  PV Array/RConn2 -- DC DC Boost Converter/LConn2
  DC AC Inverter/LConn2 -- DC DC Boost Converter/RConn2
  DC AC Inverter/RConn1 -- L/LConn1

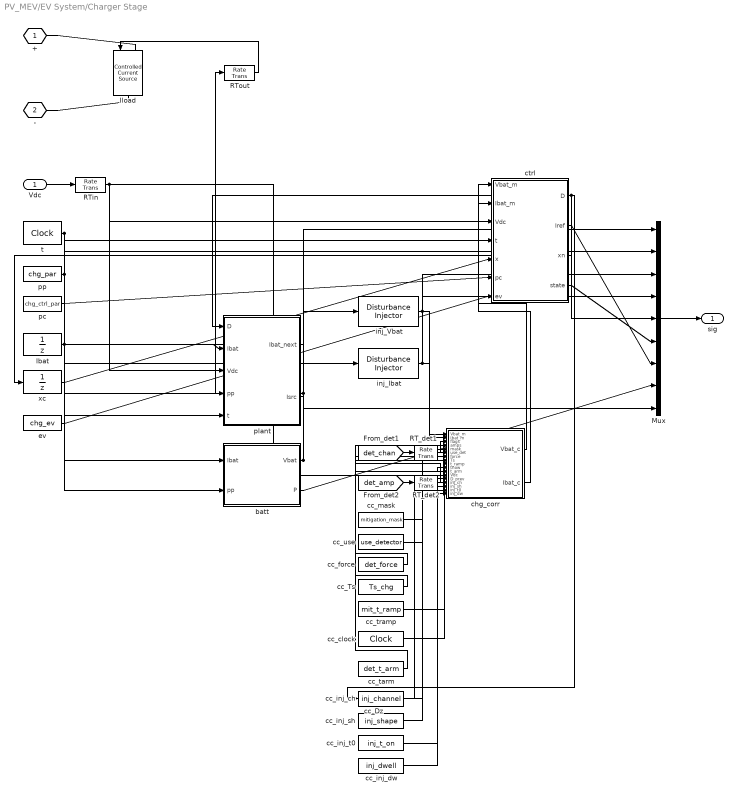
== system PV_MEV/EV System/Charger Stage ==
  Vdc : Inport
  Ibat : UnitDelay  SampleTime=Ts_chg  HasFrameUpgradeWarning=on
  Iload : spsControlledCurrentSourceLib/Controlled Current Source  Initialize=on  Source_Type=AC  Amplitude=0  Phase=0  Frequency=0  Measurements=None
  Mux : Mux  Inputs=9
  RT_det1 : RateTransition  OutPortSampleTime=Ts_chg
  RT_det2 : RateTransition  OutPortSampleTime=Ts_chg
  RTin : RateTransition  OutPortSampleTime=Ts_chg
  RTout : RateTransition  OutPortSampleTime=Ts_Power
  batt : MATLAB Function  TreatAsAtomicUnit=on
  cc_Dz : UnitDelay  SampleTime=Ts_chg  HasFrameUpgradeWarning=on
  cc_Ts : Constant  Value=Ts_chg
  cc_clock : DigitalClock  SampleTime=Ts_chg
  cc_force : Constant  Value=det_force
  cc_inj_ch : Constant  Value=inj_channel
  cc_inj_dw : Constant  Value=inj_dwell
  cc_inj_sh : Constant  Value=inj_shape
  cc_inj_t0 : Constant  Value=inj_t_on
  cc_mask : Constant  Value=mitigation_mask
  cc_tarm : Constant  Value=det_t_arm
  cc_tramp : Constant  Value=mit_t_ramp
  cc_use : Constant  Value=use_detector
  chg_corr : MATLAB Function  TreatAsAtomicUnit=on
  ctrl : MATLAB Function  TreatAsAtomicUnit=on
  ev : Constant  Value=chg_ev
  inj_Ibat : MyLibrary/Disturbance Injector  ch_id=5  Ts_inj=Ts_chg  Ts_out=Ts_chg
  inj_Vbat : MyLibrary/Disturbance Injector  ch_id=4  Ts_inj=Ts_chg  Ts_out=Ts_chg
  pc : Constant  Value=chg_ctrl_par
  plant : MATLAB Function  TreatAsAtomicUnit=on
  pp : Constant  Value=chg_par
  t : DigitalClock  SampleTime=Ts_chg
  xc : UnitDelay  InitialCondition=zeros(1,5)  SampleTime=Ts_chg  HasFrameUpgradeWarning=on
  + : PMIOPort  Side=Left
  - : PMIOPort  Port=2  Side=Left
  sig : Outport
  wires:
  Mux/1 -> sig/1
  batt/2(P) -> Mux/8
  ctrl/2(Iref) -> Mux/7
  ctrl/4(state) -> Mux/6
  RTout/1 -> Iload/1
  plant/2(Isrc) -> Mux/9, RTout/1
  ctrl/3(xn) -> xc/1
  ev/1 -> ctrl/7(ev)
  pc/1 -> ctrl/6(pc)
  xc/1 -> ctrl/5(x)
  inj_Ibat/1 -> Mux/4, chg_corr/2(Ibat_m)
  inj_Vbat/1 -> Mux/3, chg_corr/1(Vbat_m)
  batt/1(Vbat) -> Mux/1, inj_Vbat/1
  plant/1(Ibat_next) -> Ibat/1
  t/1 -> ctrl/4(t), plant/5(t)
  pp/1 -> batt/2(pp), plant/4(pp)
  RTin/1 -> ctrl/3(Vdc), plant/3(Vdc), chg_corr/12(Vdc)
  Ibat/1 -> Mux/2, inj_Ibat/1, batt/1(Ibat), plant/2(Ibat)
  ctrl/1(D) -> Mux/5, plant/1(D), cc_Dz/1
  Vdc/1 -> RTin/1
  [det_chan] -> RT_det1/1
  RT_det1/1 -> chg_corr/3(flags)
  [det_amp] -> RT_det2/1
  RT_det2/1 -> chg_corr/4(amps)
  cc_mask/1 -> chg_corr/5(mask)
  cc_use/1 -> chg_corr/6(use_det)
  cc_force/1 -> chg_corr/7(force)
  cc_Ts/1 -> chg_corr/8(Ts)
  cc_tramp/1 -> chg_corr/9(t_ramp)
  chg_corr/1(Vbat_c) -> ctrl/1(Vbat_m)
  chg_corr/2(Ibat_c) -> ctrl/2(Ibat_m)
  cc_clock/1 -> chg_corr/10(tnow)
  cc_tarm/1 -> chg_corr/11(t_arm)
  cc_Dz/1 -> chg_corr/13(D_prev)
  cc_inj_ch/1 -> chg_corr/14(inj_ch)
  cc_inj_sh/1 -> chg_corr/15(inj_sh)
  cc_inj_t0/1 -> chg_corr/16(inj_t0)
  cc_inj_dw/1 -> chg_corr/17(inj_dw)
  connections:
  -/RConn1 -- Iload/RConn1
  +/RConn1 -- Iload/LConn1

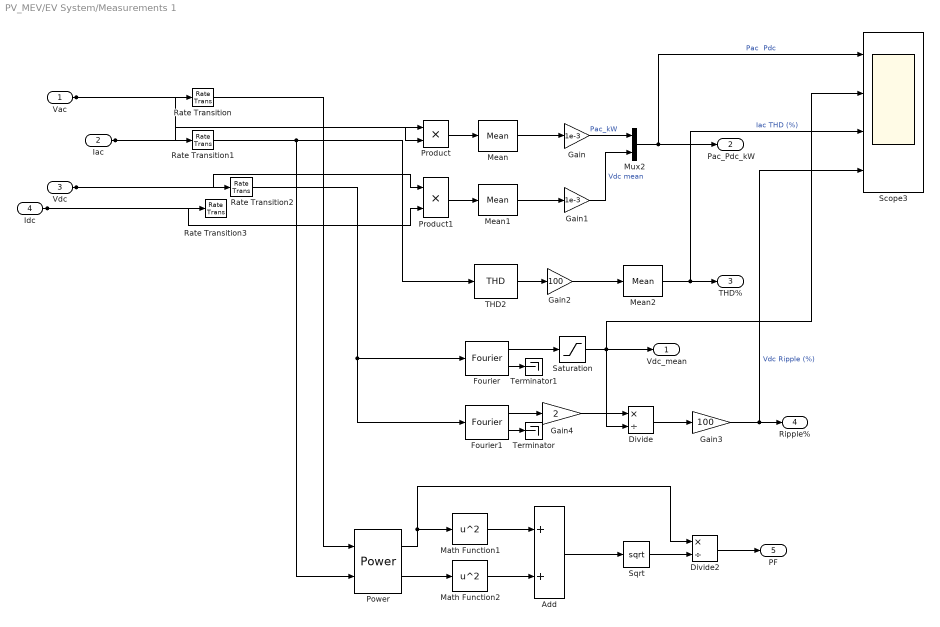
== system PV_MEV/EV System/Measurements 1 ==
  Vac : Inport
  Iac : Inport  Port=2
  Vdc : Inport  Port=3
  Idc : Inport  Port=4
  Add : Sum
  Divide : Product  Inputs=*/
  Divide2 : Product  Inputs=*/
  Fourier : spsFourierLib/Fourier  Freq=Fnom  n=0  InInit=[0, 0]  Ts=Ts_Control
  Fourier1 : spsFourierLib/Fourier  Freq=Fnom  n=2  InInit=[0, 0]  Ts=Ts_Control
  Gain : Gain  Gain=1e-3
  Gain1 : Gain  Gain=1e-3
  Gain2 : Gain  Gain=100
  Gain3 : Gain  Gain=100
  Gain4 : Gain  Gain=2
  Math Function1 : Math  Operator=square
  Math Function2 : Math  Operator=square
  Mean : spsMeanLib/Mean  Freq=Fnom  Vinit=0  Ts=Ts_Power
  Mean1 : spsMeanLib/Mean  Freq=Fnom  Vinit=0  Ts=Ts_Power
  Mean2 : spsMeanLib/Mean  Freq=Fnom  Vinit=0  Ts=Ts_Control
  Mux2 : Mux  Inputs=2
  Power : spsPowerLib/Power  Freq=Fnom  Vinit=[1, 0]  Iinit=[1, 0]  Ts=Ts_Control
  Product : Product
  Product1 : Product
  Rate Transition{,1..3} (4 alike) : RateTransition  OutPortSampleTime=Ts_Control
  Saturation : Saturate  UpperLimit=inf  LowerLimit=eps
  Scope3 : Scope  NumInputPorts=4
      settings: ActiveDisplayYMaximum=16.6658  DataLoggingSaveFormat=Array
  Sqrt : Sqrt
  THD2 : spsTHDLib/THD  Freq=Fnom  Ts=Ts_Control
  Terminator : Terminator
  Terminator1 : Terminator
  Vdc_mean : Outport
  Pac_Pdc_kW : Outport  Port=2
  THD% : Outport  Port=3
  Ripple% : Outport  Port=4
  PF : Outport  Port=5
  wires:
  Gain1/1 -> Mux2/2  "Vdc mean"
  Product1/1 -> Mean1/1
  Mean/1 -> Gain/1
  Product/1 -> Mean/1
  Gain/1 -> Mux2/1  "Pac_kW"
  THD2/1 -> Gain2/1
  Mean1/1 -> Gain1/1
  Iac/1 -> Rate Transition1/1, Product/2
  Mux2/1 -> Scope3/1, Pac_Pdc_kW/1  "Pac  Pdc"
  Gain2/1 -> Mean2/1
  Mean2/1 -> Scope3/3, THD%/1  "Iac THD (%)"
  Fourier/2 -> Terminator1/1
  Fourier/1 -> Saturation/1
  Saturation/1 -> Scope3/2, Vdc_mean/1, Divide/2
  Divide/1 -> Gain3/1
  Fourier1/1 -> Gain4/1
  Gain4/1 -> Divide/1
  Fourier1/2 -> Terminator/1
  Gain3/1 -> Scope3/4, Ripple%/1  "Vdc Ripple (%)"
  Power/1 -> Math Function1/1, Divide2/1
  Power/2 -> Math Function2/1
  Math Function1/1 -> Add/1
  Math Function2/1 -> Add/2
  Add/1 -> Sqrt/1
  Sqrt/1 -> Divide2/2
  Divide2/1 -> PF/1
  Rate Transition1/1 -> Power/2, THD2/1
  Vdc/1 -> Rate Transition2/1, Product1/1
  Idc/1 -> Rate Transition3/1, Product1/2
  Rate Transition/1 -> Power/1
  Vac/1 -> Rate Transition/1, Product/1
  Rate Transition2/1 -> Fourier/1, Fourier1/1
